simulink model "DynamixelLibrary_Prototyping"  (R2020a)
settings: Solver=FixedStepAuto  StartTime=0.0  StopTime=40  FixedStep=0.5  RelTol=1e-3  EnableMultiTasking=on
values from neighbouring files (symbols this model uses):
  serverRate = 1/10    (= 0.1)    [Run_Initializer.m]
undefined symbols (not defined in the file or in its folder): maxOmega
settings Model: SimulationMode=external  Creator=AlexC  LastModifiedBy=Kirk
settings SolverCC: PositivePriorityOrder=on
settings DataIOCC: ReturnWorkspaceOutputs=off
settings OptimizationCC: PassReuseOutputArgsThreshold=0  MaxStackSize=64  EfficientTunableParamExpr=on
settings DebuggingCC: ParameterTunabilityLossMsg=error  ArithmeticOperatorsInVariantConditions=warning
settings HardwareCC: ProdBitPerPointer=32  ProdBitPerSizeT=32  ProdBitPerPtrDiffT=32  ProdLargestAtomicInteger=Long  ProdLargestAtomicFloat=Double  ProdWordSize=32  ProdHWDeviceType=ARM Compatible->ARM Cortex
settings SFSimCC: SimUseLocalCustomCode=off  MATLABDynamicMemAlloc=off  CustomCodeUndefinedFunction=UseInterfaceOnly
settings RTWCC: SystemTargetFile=ert.tlc  HardwareBoard=Raspberry Pi  TemplateMakefile=ert_default_tmf  RTWUseLocalCustomCode=off  Toolchain=GNU GCC Raspberry Pi  BuildConfiguration=Specify  TargetLang=C++
settings CodeAppCC: ForceParamTrailComments=on  OperatorAnnotations=on
settings ERTTargetCC: CodeReplacementLibrary=GCC ARM Cortex-A8  ERTCustomFileBanners=off  SupportContinuousTime=on  SupportNonInlinedSFcns=on  RemoveResetFunc=off  SupportVariableSizeSignals=on  ModelStepFunctionPrototypeControlCompliant=off  RootIOFormat=Structure reference

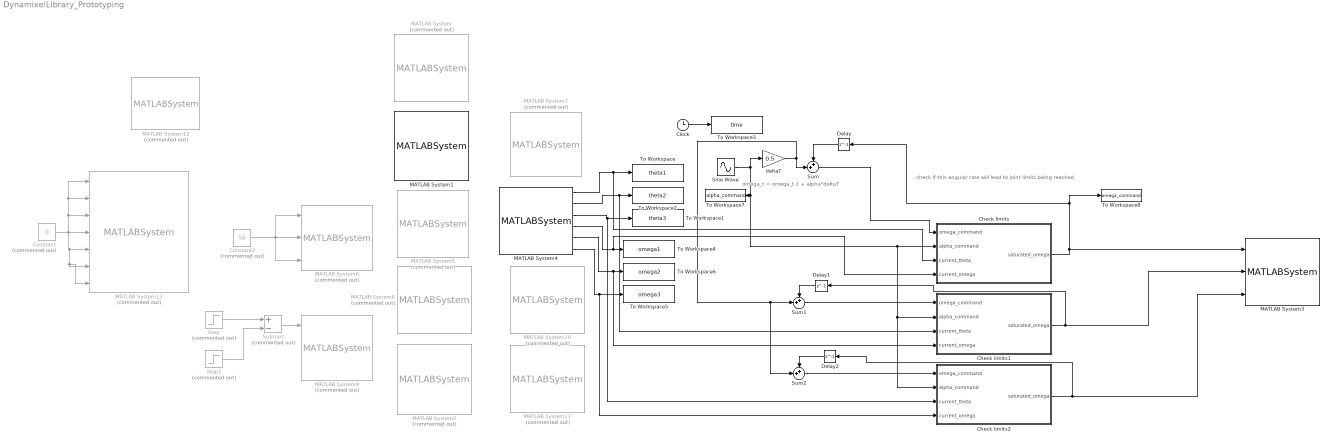
== system DynamixelLibrary_Prototyping ==
  note: check if this angular rate will lead to joint limits being reached
  note: omega_t = omega_t-1 + alpha*deltaT
  Check limits : MATLAB Function  TreatAsAtomicUnit=on
  Check limits1 : MATLAB Function  TreatAsAtomicUnit=on
  Check limits2 : MATLAB Function  TreatAsAtomicUnit=on
  Clock : Clock
  Constant : Constant  Commented=on  Value=0
  Constant2 : Constant  Commented=on  Value=50
  Delay : Delay  DelayLength=1
  Delay1 : Delay  DelayLength=1
  Delay2 : Delay  DelayLength=1
  MATLAB System : MATLABSystem  Commented=on  System=InitializeForPosition  P_GAIN=400  I_GAIN=0  D_GAIN=200  MAX_POSITION=3072  MIN_POSITION=1024  VELOCITY_PROFILE=0  ACCELERATION_PROFILE=0
      mask Type: InitializeForPosition
      mask Display: disp('InitializeForPosition');
  MATLAB System1 : MATLABSystem  System=InitializeForSpeed  P_GAIN=100  I_GAIN=1920  VELOCITY_LIMIT=22  ACCELERATION_TIME=500
      mask Type: InitializeForSpeed
      mask Display: disp('InitializeForSpeed');
  MATLAB System10 : MATLABSystem  Commented=on  System=InitializeForSpecial  CURRENT_LIMIT=850  P_GAIN=400  I_GAIN=0  D_GAIN=200  MAX_POSITION=3072  MIN_POSITION=1024  VELOCITY_LIMIT=0
      mask Type: InitializeForSpecial
      mask Display: disp('InitializeForSpecial');
  MATLAB System11 : MATLABSystem  Commented=on  System=MoveArm_Special
      mask Type: MoveArm_Special
      mask Display:
      | disp('MoveArm_Special');
      | port_label('input',1,'u1');
      | port_label('input',2,'u2');
      | port_label('input',3,'u3');
  MATLAB System12 : MATLABSystem  Commented=on  System=InitializeForArmGripper  P_GAIN_ARM=400  I_GAIN_ARM=0  D_GAIN_ARM=200  P_GAIN_PROX=400  I_GAIN_PROX=0  D_GAIN_PROX=200  P_GAIN_DIST=400  I_GAIN_DIST=0  D_GAIN_DIST=200  MAX_POSITION_ARM=3072  MIN_POSITION_ARM=1024  MAX_POSITION_PROX=3072  MIN_POSITION_PROX=1024  MAX_POSITION_DIST=3072  MIN_POSITION_DIST=1024  VELOCITY_LIMIT_ARM=0  VELOCITY_LIMIT_GRIP=0  MAX_CURRENT_GRIP=1000
      mask Type: InitializeForArmGripper
      mask Display: disp('InitializeForArmGripper');
  MATLAB System13 : MATLABSystem  Commented=on  System=MoveArmGripper_Position
      mask Type: MoveArmGripper_Position
      mask Display:
      | disp('MoveArmGripper_Position');
      | port_label('input',1,'u1');
      | port_label('input',2,'u2');
      | port_label('input',3,'u3');
      | port_label('input',4,'uL1');
      | port_label('input',5,'uR1');
      | port_label('input',6,'uL2');
      | port_label('input',7,'uR2');
  MATLAB System2 : MATLABSystem  Commented=on  System=MoveArm_Position
      mask Type: MoveArm_Position
      mask Display:
      | disp('MoveArm_Position');
      | port_label('input',1,'u1');
      | port_label('input',2,'u2');
      | port_label('input',3,'u3');
  MATLAB System3 : MATLABSystem  System=MoveArm_Speed
      mask Type: MoveArm_Speed
      mask Display:
      | disp('MoveArm_Speed');
      | port_label('input',1,'u1');
      | port_label('input',2,'u2');
      | port_label('input',3,'u3');
  MATLAB System4 : MATLABSystem  System=ReadArm_Position_Rates  SampleTime=0.5
      mask Type: ReadArm_Position_Rates
      mask Display:
      | disp('ReadArm_Position_Rates');
      | port_label('output',1,'theta1');
      | port_label('output',2,'theta2');
      | port_label('output',3,'theta3');
      | port_label('output',4,'omega1');
      | port_label('output',5,'omega2');
      | port_label('output',6,'omega3');
  MATLAB System5 : MATLABSystem  Commented=on  System=InitializeForPWM  PWM_LIMIT=885
      mask Type: InitializeForPWM
      mask Display: disp('InitializeForPWM');
  MATLAB System6 : MATLABSystem  Commented=on  System=MoveArm_PWM
      mask Type: MoveArm_PWM
      mask Display:
      | disp('MoveArm_PWM');
      | port_label('input',1,'u1');
      | port_label('input',2,'u2');
      | port_label('input',3,'u3');
  MATLAB System7 : MATLABSystem  Commented=on  System=ReadArm_Load  SampleTime=0.1
      mask Type: ReadArm_Load
      mask Display:
      | disp('ReadArm_Load');
      | port_label('output',1,'y1');
      | port_label('output',2,'y2');
      | port_label('output',3,'y3');
  MATLAB System8 : MATLABSystem  Commented=on  System=InitializeForTorque  CURRENT_LIMIT=850
      mask Type: InitializeForTorque
      mask Display: disp('InitializeForTorque');
  MATLAB System9 : MATLABSystem  Commented=on  System=MoveArm_Torque
      mask Type: MoveArm_Torque
      mask Display:
      | disp('MoveArm_Torque');
      | port_label('input',1,'u1');
      | port_label('input',2,'u2');
      | port_label('input',3,'u3');
      | port_label('output',1,'y1');
      | port_label('output',2,'y2');
      | port_label('output',3,'y3');
  Sine Wave : Sin  Amplitude=0.1  Frequency=2*pi/40  Phase=pi/2  SampleTime=0.5
  Step : Step  Commented=on  Time=5  After=30  SampleTime=0
  Step1 : Step  Commented=on  Time=6  After=30  SampleTime=0
  Subtract : Sum  Commented=on  Inputs=+-
  Sum : Sum  Inputs=++|
  Sum1 : Sum  Inputs=++|
  Sum2 : Sum  Inputs=++|
  To Workspace : ToWorkspace  VariableName=theta1  SampleTime=-1
      settings: Save2DSignal=2-D array (concatenate along first dimension)
  To Workspace1 : ToWorkspace  VariableName=theta3  SampleTime=-1
      settings: Save2DSignal=2-D array (concatenate along first dimension)
  To Workspace2 : ToWorkspace  VariableName=theta2  SampleTime=-1
      settings: Save2DSignal=2-D array (concatenate along first dimension)
  To Workspace3 : ToWorkspace  VariableName=time  SampleTime=-1
  To Workspace4 : ToWorkspace  VariableName=omega1  SampleTime=-1
      settings: Save2DSignal=2-D array (concatenate along first dimension)
  To Workspace5 : ToWorkspace  VariableName=omega3  SampleTime=-1
      settings: Save2DSignal=2-D array (concatenate along first dimension)
  To Workspace6 : ToWorkspace  VariableName=omega2  SampleTime=-1
      settings: Save2DSignal=2-D array (concatenate along first dimension)
  To Workspace7 : ToWorkspace  VariableName=alpha_command  SampleTime=-1
  To Workspace8 : ToWorkspace  VariableName=omega_command  SampleTime=-1
  deltaT : Gain  Gain=0.5
  wires:
  Constant2/1 -> MATLAB System6/3, MATLAB System6/1, MATLAB System6/2
  Step/1 -> Subtract/1
  Step1/1 -> Subtract/2
  Subtract/1 -> MATLAB System9/1
  Constant/1 -> MATLAB System13/7, MATLAB System13/6, MATLAB System13/5, MATLAB System13/3, MATLAB System13/2, MATLAB System13/1, MATLAB System13/4
  MATLAB System4/1 -> Check limits/3(current_theta), To Workspace/1
  MATLAB System4/2 -> Check limits1/3(current_theta), To Workspace2/1
  MATLAB System4/3 -> To Workspace1/1, Check limits2/3(current_theta)
  Clock/1 -> To Workspace3/1
  MATLAB System4/4 -> Check limits/4(current_omega), To Workspace4/1
  MATLAB System4/5 -> Check limits1/4(current_omega), To Workspace6/1
  MATLAB System4/6 -> Check limits2/4(current_omega), To Workspace5/1
  Sine Wave/1 -> deltaT/1, Check limits2/2(alpha_command), Check limits1/2(alpha_command), Check limits/2(alpha_command), To Workspace7/1
  Check limits/1(saturated_omega) -> To Workspace8/1, Delay/1, MATLAB System3/1
  Sum/1 -> Check limits/1(omega_command)
  deltaT/1 -> Sum/2, Sum2/2, Sum1/2
  Delay/1 -> Sum/1
  Check limits1/1(saturated_omega) -> Delay1/1, MATLAB System3/2
  Check limits2/1(saturated_omega) -> Delay2/1, MATLAB System3/3
  Delay1/1 -> Sum1/1
  Delay2/1 -> Sum2/1
  Sum1/1 -> Check limits1/1(omega_command)
  Sum2/1 -> Check limits2/1(omega_command)

== matlab function DynamixelLibrary_Prototyping/Check limits1 ==
  data: omega_command input; alpha_command input; current_theta input; saturated_omega output; current_omega input; serverRate parameter; maxOmega parameter
function saturated_omega = check_limits(omega_command, alpha_command, current_theta, current_omega, serverRate, maxOmega)

buffer_angle = 0; % [deg]
next_theta = current_theta + current_omega * (serverRate) + 0.5 * alpha_command * (serverRate) ^2;

if (((next_theta >= pi/2 - buffer_angle*pi/180) && (omega_command > 0)) || ((next_theta <= -pi/2 + buffer_angle*pi/180) && (omega_command < 0)))
    saturated_omega = 0;
elseif omega_command > maxOmega
    saturated_omega = maxOmega;
elseif omega_command < - maxOmega
    saturated_omega = -maxOmega;
else
    saturated_omega = omega_command;
end

== matlab function DynamixelLibrary_Prototyping/Check limits ==
  data: omega_command input; alpha_command input; current_theta input; saturated_omega output; current_omega input; serverRate parameter; maxOmega parameter
function saturated_omega = check_limits(omega_command, alpha_command, current_theta, current_omega, serverRate, maxOmega)

buffer_angle = 0; % [deg]
next_theta = current_theta + current_omega * (serverRate) + 0.5 * alpha_command * (serverRate) ^2;

if (((next_theta >= pi/2 - buffer_angle*pi/180) && (omega_command > 0)) || ((next_theta <= -pi/2 + buffer_angle*pi/180) && (omega_command < 0)))
    saturated_omega = 0;
elseif omega_command > maxOmega
    saturated_omega = maxOmega;
elseif omega_command < - maxOmega
    saturated_omega = -maxOmega;
else
    saturated_omega = omega_command;
end

== matlab function DynamixelLibrary_Prototyping/Check limits2 ==
  data: omega_command input; alpha_command input; current_theta input; saturated_omega output; current_omega input; serverRate parameter; maxOmega parameter
function saturated_omega = check_limits(omega_command, alpha_command, current_theta, current_omega, serverRate, maxOmega)

buffer_angle = 0; % [deg]
next_theta = current_theta + current_omega * (serverRate) + 0.5 * alpha_command * (serverRate) ^2;

if (((next_theta >= pi/2 - buffer_angle*pi/180) && (omega_command > 0)) || ((next_theta <= -pi/2 + buffer_angle*pi/180) && (omega_command < 0)))
    saturated_omega = 0;
elseif omega_command > maxOmega
    saturated_omega = maxOmega;
elseif omega_command < - maxOmega
    saturated_omega = -maxOmega;
else
    saturated_omega = omega_command;
end
